simulink model "Slam_part"  (R2024a)
settings: Solver=VariableStepAuto  StartTime=0.0  StopTime=inf  RelTol=1e-3
libraries: robotcorelib x2
settings Model: Creator=user  LastModifiedBy=user

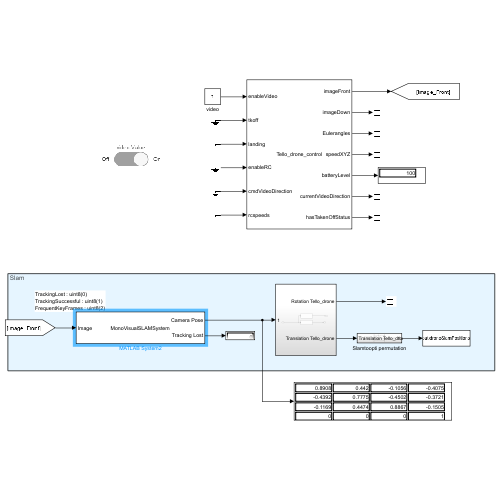
[thumbnail: Simulink's stored preview of the top-level diagram]
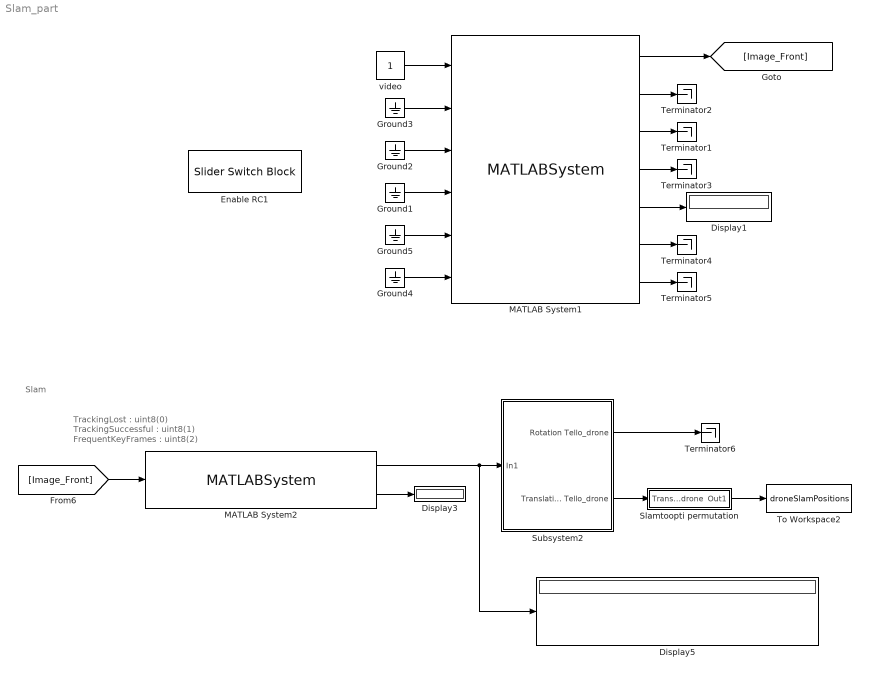
== system Slam_part ==
  note: Slam
  note: TrackingLost : uint8(0)
      | TrackingSuccessful : uint8(1)
      | FrequentKeyFrames : uint8(2)
  Display1 : Display
  Display3 : Display
  Display5 : Display
  Enable RC1 : SliderSwitchBlock
      settings: Values={{'Off', 'On'}, [0 1]}
  Ground{1..5} (5 alike) : Ground
  MATLAB System1 : MATLABSystem  System=Tello_drone_control  droneIP=127.0.0.1  SimulateUsing=Interpreted execution
      mask Type: Tello_drone_control
      mask Display:
      | disp('Tello_drone_control');
      | port_label('input',1,'enableVideo');
      | port_label('input',2,'tkoff');
      | port_label('input',3,'landing');
      | port_label('input',4,'enableRC');
      | port_label('input',5,'cmdVideoDirection');
      | port_label('input',6,'rcspeeds');
      | port_label('output',1,'imageFront');
      | port_label('output',2,'imageDown');
      | port_label('output',3,'Eulerangles');
      | port_label('output',4,'speedXYZ');
      | port_label('output',5,'batteryLevel');
      | port_label('output',6,'currentVideoDirection');
      | port_label('output',7,'hasTakenOffStatus');
  MATLAB System2 : MATLABSystem  System=MonoVisualSLAMSystem  FocalLength=[ 894, 896]  PrincipalPoint=[490,355.6]  ImageSize=[ 720, 960 ]  numPoints=800  numSkipFrames=15  SimulateUsing=Code generation
      mask Type: MonoVisualSLAMSystem
      mask Display:
      | disp('MonoVisualSLAMSystem');
      | port_label('input',1,'Image');
      | port_label('output',1,'Camera Pose');
      | port_label('output',2,'Tracking Lost');
  Slamtoopti permutation : Subsystem
  Subsystem2 : Subsystem
  Terminator{1..6} (6 alike) : Terminator
  To Workspace2 : ToWorkspace  VariableName=droneSlamPositions  SampleTime=-1
  video : Constant
  wires:
  [Image_Front] -> MATLAB System2/1
  Slamtoopti permutation/1(Out1) -> To Workspace2/1
  MATLAB System2/2 -> Display3/1
  MATLAB System2/1 -> Display5/1, Subsystem2/1(In1)
  Subsystem2/1(Rotation Tello_drone) -> Terminator6/1
  Subsystem2/2(Translation Tello_drone) -> Slamtoopti permutation/1(Translation Tello_drone)
  Ground3/1 -> MATLAB System1/2
  MATLAB System1/1 -> [Image_Front]
  MATLAB System1/6 -> Terminator4/1
  Ground1/1 -> MATLAB System1/4
  Ground5/1 -> MATLAB System1/5
  MATLAB System1/4 -> Terminator3/1
  MATLAB System1/2 -> Terminator2/1
  MATLAB System1/7 -> Terminator5/1
  video/1 -> MATLAB System1/1
  MATLAB System1/5 -> Display1/1
  Ground2/1 -> MATLAB System1/3
  MATLAB System1/3 -> Terminator1/1
  Ground4/1 -> MATLAB System1/6

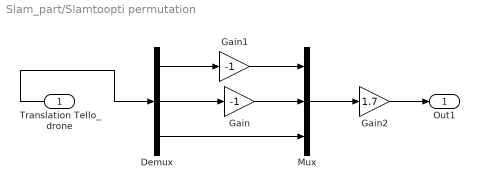
== system Slam_part/Slamtoopti permutation ==
  Translation Tello_drone : Inport
  Demux : Demux  Outputs=3
  Gain : Gain  Gain=-1
  Gain1 : Gain  Gain=-1
  Gain2 : Gain  Gain=1.7
  Mux : Mux  Inputs=3
  Out1 : Outport
  wires:
  Demux/2 -> Gain/1
  Demux/1 -> Gain1/1
  Mux/1 -> Gain2/1
  Gain/1 -> Mux/2
  Demux/3 -> Mux/3
  Gain1/1 -> Mux/1
  Gain2/1 -> Out1/1
  Translation Tello_drone/1 -> Demux/1

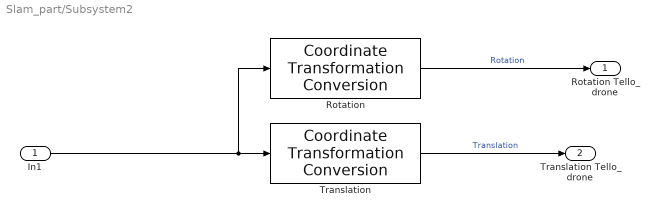
== system Slam_part/Subsystem2 ==
  In1 : Inport
  Rotation : robotcorelib/Coordinate Transformation Conversion  InputRepresentation=Homogeneous Transformation  InputEulerSequence=ZYX  ShowTrVecInputPort=on  OutputRepresentation=Rotation Matrix  OutputEulerSequence=ZYX  ShowTrVecOutputPort=off  SimulateUsing=Code generation
      settings: LibrarySourceBlock=uavutilslib/Coordinate Transformation Conversion
  Translation : robotcorelib/Coordinate Transformation Conversion  InputRepresentation=Homogeneous Transformation  InputEulerSequence=ZYX  ShowTrVecInputPort=on  OutputRepresentation=Translation Vector  OutputEulerSequence=ZYX  ShowTrVecOutputPort=on  SimulateUsing=Code generation
      settings: LibrarySourceBlock=uavutilslib/Coordinate Transformation Conversion
  Rotation Tello_drone : Outport
  Translation Tello_drone : Outport  Port=2
  wires:
  Translation/1 -> Translation Tello_drone/1  "Translation"
  Rotation/1 -> Rotation Tello_drone/1  "Rotation"
  In1/1 -> Rotation/1, Translation/1
